simulink model "fixed_lqr"  (R2025b)
settings: Solver=ode45  StartTime=0.0  StopTime=3  MaxStep=0.005  RelTol=1e-3
InitFcn:
  | addpath(fileparts(get_param(bdroot, 'FileName')))
settings Model: Creator=derekg  LastModifiedBy=derekg

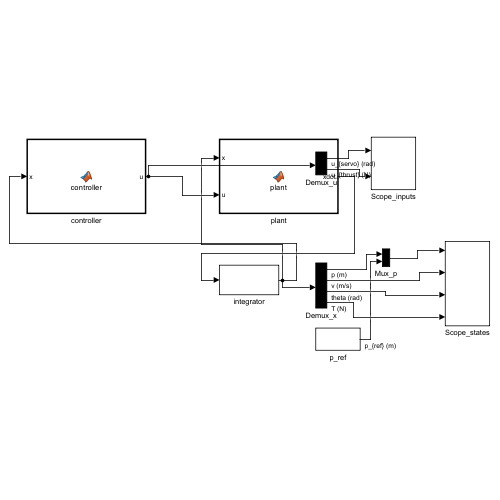
[thumbnail: Simulink's stored preview of the top-level diagram]
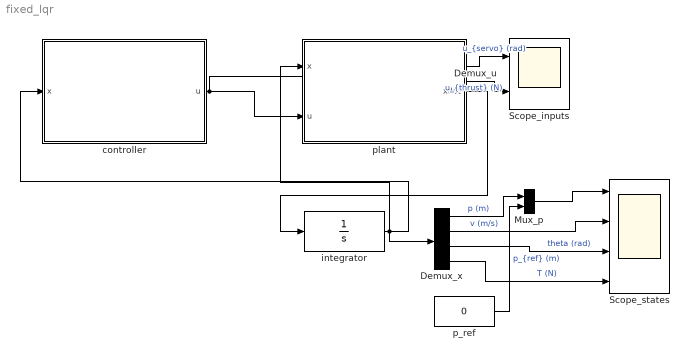
== system fixed_lqr ==
  Demux_u : Demux  Outputs=2
  Demux_x : Demux
  Mux_p : Mux  Inputs=2
  Scope_inputs : Scope  NumInputPorts=2
  Scope_states : Scope  NumInputPorts=4
  controller : MATLAB Function  TreatAsAtomicUnit=on
  integrator : Integrator  InitialCondition=[0.15; 0; 0; 2.574]
  p_ref : Constant  Value=0
  plant : MATLAB Function  TreatAsAtomicUnit=on
  wires:
  integrator/1 -> controller/1(x), plant/1(x), Demux_x/1
  controller/1(u) -> plant/2(u), Demux_u/1
  plant/1(xdot) -> integrator/1
  Demux_x/3 -> Scope_states/3  "theta (rad)"
  Demux_x/1 -> Mux_p/1  "p (m)"
  p_ref/1 -> Mux_p/2  "p_{ref} (m)"
  Mux_p/1 -> Scope_states/1
  Demux_x/2 -> Scope_states/2  "v (m/s)"
  Demux_x/4 -> Scope_states/4  "T (N)"
  Demux_u/1 -> Scope_inputs/1  "u_{servo} (rad)"
  Demux_u/2 -> Scope_inputs/2  "u_{thrust} (N)"

== matlab function fixed_lqr/controller ==
  data: x input; u output
function u = controller(x)
% Fixed-gain LQR. Single operating point: theta*=0, T*=T_r_nom.
% Control law: u = u_star - K_fixed * (x - x_star)
persistent K_fixed x_star u_star
if isempty(K_fixed)
    tmp    = coder.load('gain_schedule_tier1.mat');
    K_fixed = tmp.K_fixed;
    x_star  = tmp.x_star;
    u_star  = tmp.u_star;
end
u = u_star - K_fixed * (x - x_star);
u(1) = max(min(u(1), pi/3), -pi/3);  % servo ±60°
u(2) = max(min(u(2), 4.17), 0);      % thrust 0–4.17 N (static sweep at 1950 µs)
end

== matlab function fixed_lqr/plant ==
  data: x input; u input; xdot output
function xdot = plant(x, u)
% Nonlinear EOM: x = [p; v; theta; T],  u = [theta_cmd_rad; T_cmd_N]
m          = 0.4536;
tau_servo  = 0.0244;
tau_thrust = 0.0781;
mu_c       = 0.8158;
v_sign = tanh(x(2) / 0.05);   % smooth sign: avoids chattering at v≈0 (ε = 5 mm/s)
xdot = [x(2);
        (x(4)*sin(x(3)) - mu_c*v_sign) / m;
        (u(1) - x(3)) / tau_servo;
        (u(2) - x(4)) / tau_thrust];
end
